simulink model "myKalmanFilter"  (R2018b)
settings: Solver=FixedStepAuto  StartTime=0.0  StopTime=sim_time  FixedStep=0.01  RelTol=1e-3
settings Model: Creator=gizem  LastModifiedBy=gizem

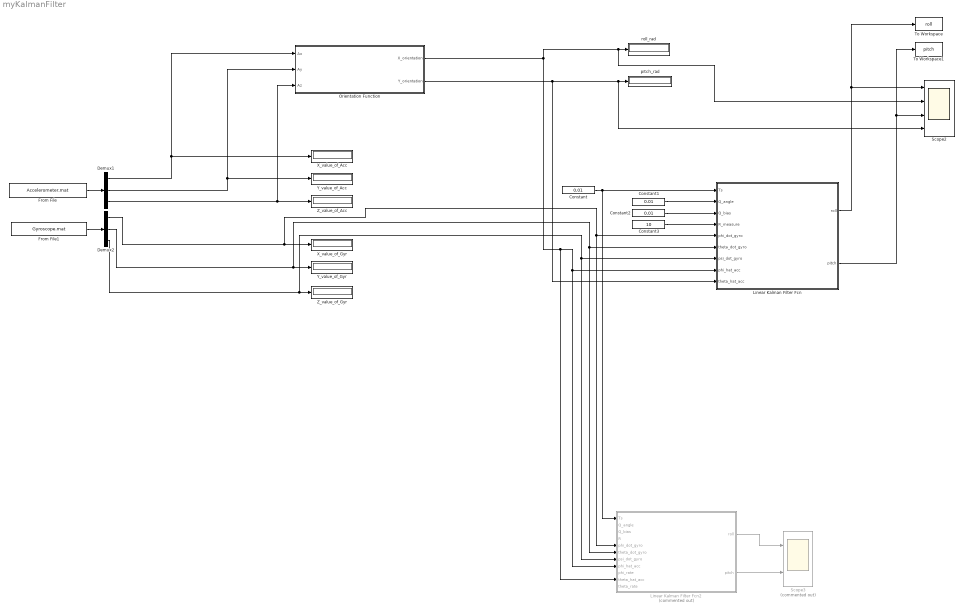
== system myKalmanFilter ==
  Constant : Constant  Value=0.01
  Constant1 : Constant  Value=0.01
  Constant2 : Constant  Value=0.01
  Constant3 : Constant  Value=10
  Demux1 : Demux  Outputs=3
  Demux2 : Demux  Outputs=3
  From File : FromFile  FileName=Accelerometer.mat  SampleTime=0.01
  From File1 : FromFile  FileName=Gyroscope.mat  SampleTime=0.01
  Linear Kalman Filter Fcn : MATLAB Function  TreatAsAtomicUnit=on
  Linear Kalman Filter Fcn2 : MATLAB Function  Commented=on  TreatAsAtomicUnit=on
  Orientation Function : MATLAB Function  TreatAsAtomicUnit=on
  Scope2 : Scope  NumInputPorts=4
  Scope3 : Scope  Commented=on  NumInputPorts=2
  To Workspace : ToWorkspace  VariableName=roll  SaveFormat=Timeseries  SampleTime=-1
  To Workspace1 : ToWorkspace  VariableName=pitch  SaveFormat=Timeseries  SampleTime=-1
  X_value_of_Acc : Display
      settings: Format=bank  Decimation=4
  X_value_of_Gyr : Display
      settings: Format=bank
  Y_value_of_Acc : Display
      settings: Format=bank
  Y_value_of_Gyr : Display
      settings: Format=bank
  Z_value_of_Acc : Display
      settings: Format=bank
  Z_value_of_Gyr : Display
      settings: Format=bank
  pitch_rad : Display
  roll_rad : Display
      settings: Format=bank
  wires:
  Orientation Function/2(Y_orientation) -> Linear Kalman Filter Fcn/9(theta_hat_acc), Scope2/4, pitch_rad/1
  From File/1 -> Demux1/1
  From File1/1 -> Demux2/1
  Demux1/3 -> Orientation Function/3(Az), Z_value_of_Acc/1
  Demux1/2 -> Orientation Function/2(Ay), Y_value_of_Acc/1
  Demux1/1 -> Orientation Function/1(Ax), X_value_of_Acc/1
  Orientation Function/1(X_orientation) -> Scope2/2, roll_rad/1, Linear Kalman Filter Fcn2/10(theta_hat_acc), Linear Kalman Filter Fcn2/8(phi_hat_acc), Linear Kalman Filter Fcn/8(phi_hat_acc)
  Constant/1 -> Linear Kalman Filter Fcn2/1(Ts), Linear Kalman Filter Fcn/1(Ts)
  Linear Kalman Filter Fcn/1(roll) -> Scope2/1, To Workspace/1
  Linear Kalman Filter Fcn2/1(roll) -> Scope3/1
  Linear Kalman Filter Fcn2/2(pitch) -> Scope3/2
  Linear Kalman Filter Fcn/2(pitch) -> To Workspace1/1, Scope2/3
  Demux2/1 -> Linear Kalman Filter Fcn2/5(phi_dot_gyro), Linear Kalman Filter Fcn/5(phi_dot_gyro), X_value_of_Gyr/1
  Demux2/2 -> Linear Kalman Filter Fcn2/6(theta_dot_gyro), Linear Kalman Filter Fcn/6(theta_dot_gyro), Y_value_of_Gyr/1
  Demux2/3 -> Linear Kalman Filter Fcn2/7(psi_dot_gyro), Linear Kalman Filter Fcn/7(psi_dot_gyro), Z_value_of_Gyr/1
  Constant1/1 -> Linear Kalman Filter Fcn/2(Q_angle)
  Constant2/1 -> Linear Kalman Filter Fcn/3(Q_bias)
  Constant3/1 -> Linear Kalman Filter Fcn/4(R_measure)

== matlab function myKalmanFilter/Linear Kalman Filter Fcn2 ==
  data: Ts input; Q_angle input; Q_bias input; R input; phi_dot_gyro input; theta_dot_gyro input; psi_dot_gyro input; phi_hat_acc input; phi_rate input; roll output; theta_hat_acc input; pitch output; theta_rate input
% Algorithm -- implimentation of Linear-Kalman filter for a 6-DOF IMU using
% a single axis for testing. A single axis consisting of both anaccelerometer
% input and gyroscope input from IMU.
% Author: RM van Rensburg
% for IMU testing purposes
% Date: 26-04-2015
% Version: 1.0,tested on Matlab R2015a

% phi = roll(p) -> x
% theta = pitch(q) -> y
% psi = yaw(r) -> z

function [roll, pitch] = myKalmanFilter2(Ts,...
                                         Q_angle,Q_bias,R,...
                                         phi_dot_gyro, theta_dot_gyro, psi_dot_gyro,...
                                         phi_hat_acc, phi_rate,...
                                         theta_hat_acc,...
                                         theta_rate)
                      
    % Process noise covariance matrix  
    A = [1 -Ts 0 0; 0 1 0 0; 0 0 1 -Ts; 0 0 0 1];
    B = [Ts 0 0 0; 0 0 Ts 0]';
    C = [1 0 0 0; 0 0 1 0];
    Q = [Q_angle 0 0 0; 0 Q_bias 0 0; 0 0 Q_angle 0; 0 0 0 Q_bias]*Ts;
    state_estimate = [0 0 0 0]';

    p = phi_dot_gyro;
    q = theta_dot_gyro;
    r = psi_dot_gyro;

    % init
    persistent phi_hat_;
    if isempty(phi_hat_);phi_hat_ = 0;
    else phi_hat_ = state_estimate(1);
    end

    persistent bias_phi_hat_;
    if isempty(bias_phi_hat_);bias_phi_hat_ = 0;
    else state_estimate(2) = bias_phi_hat_; 
    end
%     bias_phi_hat_= bias_phi_hat;

    persistent theta_hat_;
    if isempty(theta_hat_);theta_hat_ = 0;
    else state_estimate(3) = theta_hat_; 
    end
%     theta_hat_= theta_hat;

    persistent bias_theta_hat_;
    if isempty(bias_theta_hat_);bias_theta_hat_ = 0;
    else state_estimate(4) = bias_theta_hat_; 
    end
%     bias_theta_hat_= bias_theta_hat;

    phi_dot   = p + sin(phi_hat_) * tan(theta_hat_) * q + cos(phi_hat_) * tan(theta_hat_) * r;
    theta_dot = cos(phi_hat_) * q - sin(phi_hat_) * r;

    % Predict
    state_estimate = A * state_estimate + B * [phi_dot, theta_dot]';
    persistent P_;
    if isempty(P_);P_ = eye(4); 
    else P_ = A * P_ * A' + Q;
    end

    % Update
    measurement = [phi_hat_acc theta_hat_acc]';
    y_tilde = measurement - C * state_estimate;
    S = R + C * P_ * C';
    K = P_ * C' * (S^-1);
    state_estimate = state_estimate + K * y_tilde;
    P_ = (eye(4) - K * C) * P_;
    
    P = P_;
%     phi_hat_ = state_estimate(1);
%     bias_phi_hat_ = state_estimate(2);
%     theta_hat_ = state_estimate(3);
%     bias_theta_hat_ = state_estimate(4);
    
    roll = phi_hat_;
    pitch = theta_hat_;   
    
return

end

== matlab function myKalmanFilter/Linear Kalman Filter Fcn ==
  data: Ts input; Q_angle input; Q_bias input; R_measure input; phi_dot_gyro input; theta_dot_gyro input; psi_dot_gyro input; phi_hat_acc input; roll output; theta_hat_acc input; pitch output
% phi = roll(p) -> x
% theta = pitch(q) -> y
% psi = yaw(r) -> z

function [roll, pitch] = myKalmanFilter(Ts, Q_angle, Q_bias, R_measure, phi_dot_gyro, theta_dot_gyro, psi_dot_gyro, phi_hat_acc, theta_hat_acc)
                      
    % Process noise covariance matrix  
    A = [1 -Ts 0 0; 0 1 0 0; 0 0 1 -Ts; 0 0 0 1];
    B = [Ts 0 0 0; 0 0 Ts 0]';
    C = [1 0 0 0; 0 0 1 0];
    Q = [Q_angle 0 0 0 ; 0 Q_bias 0 0; 0 0 Q_angle 0; 0 0 0 Q_bias];
    R = eye(2) * R_measure;
    

    % init
    
    persistent state_estimate;
    if isempty(state_estimate);state_estimate = [0 0 0 0]';
    end
    
    persistent phi_hat_;
    if isempty(phi_hat_);phi_hat_ = 1.5;
    end

    persistent bias_phi_hat_;
    if isempty(bias_phi_hat_);bias_phi_hat_ = 0;
    end
%     bias_phi_hat_= bias_phi_hat;

    persistent theta_hat_;
    if isempty(theta_hat_);theta_hat_ = 1.5;
    end
    
    persistent bias_theta_hat_;
    if isempty(bias_theta_hat_);bias_theta_hat_ = 0;
    end
    
    p = phi_dot_gyro - bias_phi_hat_;
    q = theta_dot_gyro - bias_theta_hat_;
    r = psi_dot_gyro;

    %rotation applied. really needed?
    phi_dot   = p + sin(phi_hat_) * tan(theta_hat_) * q + cos(phi_hat_) * tan(theta_hat_) * r;
    theta_dot = cos(phi_hat_) * q - sin(phi_hat_) * r;

%     phi_dot   = p;
%     theta_dot = q;

    
    % Predict
    state_estimate = A * state_estimate + B * [phi_dot, theta_dot]';

    persistent P_;
    if isempty(P_)
        P_ = eye(4); 
    else
        P_ = A * P_ * A' + Q;
    end

    % Update
    measurement = [phi_hat_acc theta_hat_acc]';
    y_tilde = measurement - C * state_estimate;
    S = R + C * P_ * C';
    K = P_ * C' * (S^-1);
    state_estimate = state_estimate + K * y_tilde;
    P = (eye(4) - K * C) * P_;
       
    phi_hat_ = state_estimate(1);
    bias_phi_hat_ = state_estimate(2);
    theta_hat_ = state_estimate(3);
    bias_theta_hat_ = state_estimate(4);
    
    P_ = P;
    
    roll = phi_hat_;
    pitch = theta_hat_;   
    
return

end

== matlab function myKalmanFilter/Orientation Function ==
  data: Ax input; X_orientation output; Y_orientation output; Ay input; Az input
% Computing orientation of tri-axial acclerometer data from IMU 
% Author: RM van Rensburg
% Date: 26-04-2015
% Version: 1.0,tested on Matlab R2015a

function [X_orientation,...
          Y_orientation]...
          = OrientationFcn(Ax,Ay,Az)
     
      
% Using x and y from accelerometer (g-forces), calculate x and y angles
% Data directly obtained from IMU
% Using the following formulae
% Ax = arctan{X/sqrt(Y*Y + Z*Z)}
% Ay = arctan{Y/sqrt(X*X + Z*Z)}

X_orientation   = atan2(Ay, sqrt(Ax ^ 2 + Az ^ 2));
Y_orientation = atan2(-Ax, sqrt(Ay ^ 2 + Az ^ 2));

% % Computing the X*X, Y*Y, Z*Z
% X2 = power(X_value_of_Acc,2);
% Y2 = power(Y_value_of_Acc,2);
% Z2 = power(Z_value_of_Acc,2);
% 
% % x-axis angle
% result = sqrt(Y2 + Z2);
% result = X_value_of_Acc / result;
% x_angle_rad = atan(result);
% X_orientation_of_Acc = x_angle_rad;
% % X_orientation_of_Acc = (x_angle_rad * 180) / pi;
% 
% % y-axis angle
% result = sqrt(X2 + Z2);
% result = Y_value_of_Acc / result;
% y_angle_rad = atan(result);
% Y_orientation_of_Acc = y_angle_rad;
% % Y_orientation_of_Acc = (y_angle_rad * 180) / pi;

% z-axis angle - cant be calculated with this method
% result = sqrt(Y2 + X2);
% result = Z_value_of_Acc / result;
% z_angle_rad = atan(result);
% Z_orientation_of_Acc = (z_angle_rad * 180) / pi;

end
